simulink model "sampleModel1661"  (R2023a)
settings: Solver=VariableStepAuto  StartTime=0.0  StopTime=10.0  RelTol=1e-3
libraries: hdlsllib x5, simulink x2
settings Model: Creator=user1  LastModifiedBy=user1

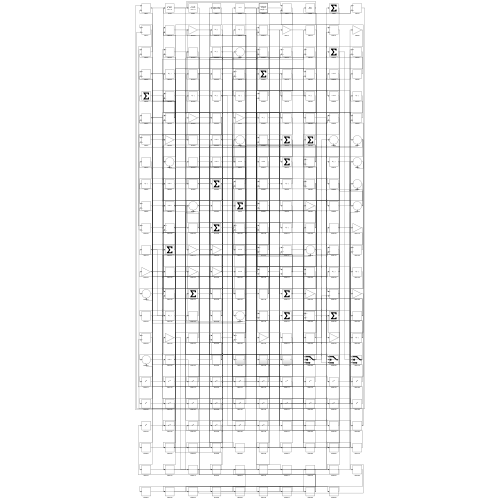
[thumbnail: Simulink's stored preview of the top-level diagram]
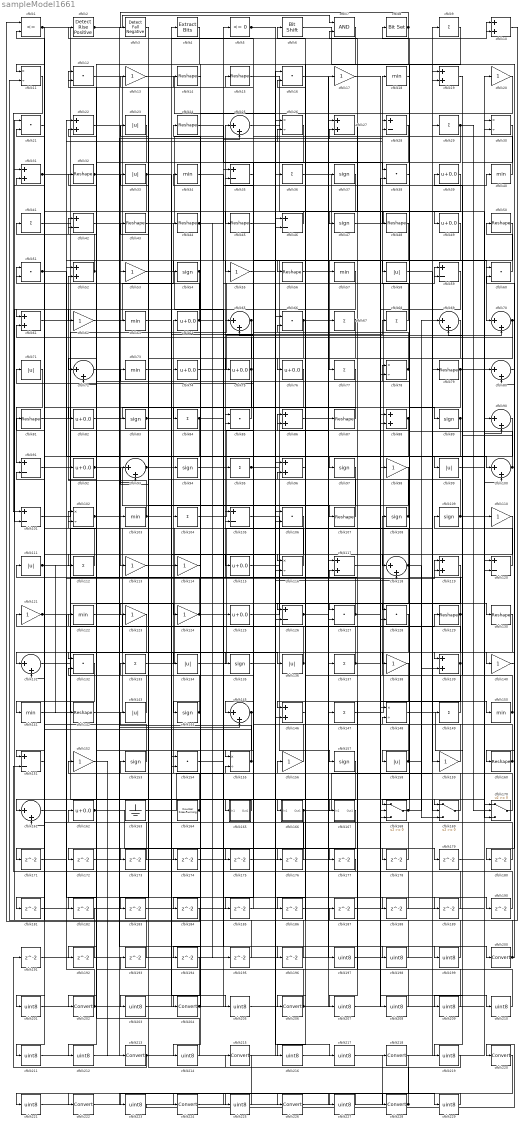
== system sampleModel1661 ==
  cfblk1 : RelationalOperator  Operator=<=  OutDataTypeStr=boolean  InputSameDT=off
  cfblk{10,19,22,27,31,52,61,86,88,96,117,119,139,146} (14 alike) : Sum
  cfblk{25,65,69..70,72,80,90,93,100,118,131,145,161} (13 alike) : Sum  Inputs=|++
  cfblk{28,35,42,46,59,91,101,105,120,126,151} (11 alike) : Sum  Inputs=+-
  cfblk{11,26,30,78,102,116,148,155} (8 alike) : Product  Inputs=*/  RndMeth=Zero  SaturateOnIntegerOverflow=on
  cfblk{18,34,40,57,63,73,103,122,141,150} (10 alike) : MinMax
  cfblk{9,29,36,41,67..68,77,84,95,104,112,133,137,147,149} (15 alike) : Sum  Inputs=+
  cfblk{12,16,21,38,51,60,66,85,106,127..128,132,154} (13 alike) : DotProduct  OutDataTypeStr=Inherit: Inherit via internal rule
  cfblk{14..15,24,32,43..45,48,50,56,79,81,87,107,129..130,142,160} (18 alike) : Reshape
  cfblk{37,47,54,83,89,94,97,108..109,135,144,153,157} (13 alike) : Signum
  cfblk{13,17,20,53,55,62,98,110,113..114,121,123..124,138,140,152,156,159} (18 alike) : Gain
  cfblk{23,33,58,71,99,111,134,136,143,158} (10 alike) : Abs  SaturateOnIntegerOverflow=off
  cfblk{39,49,64,74..76,82,92,115,125,162} (11 alike) : Bias  Bias=0.0  SaturateOnIntegerOverflow=off
  cfblk163 : Ground
  cfblk164 : hdlsllib/Sources/Counter Free-Running  NumBits=16  tsamp=-1
  cfblk165 : Subsystem
      settings: LibrarySourceBlock=|
      | hdlsllib/Ports &
      | Subsystems/Subsystem
  cfblk166 : Subsystem
      settings: LibrarySourceBlock=|
      | hdlsllib/Ports &
      | Subsystems/Subsystem
  cfblk167 : Subsystem
      settings: LibrarySourceBlock=|
      | hdlsllib/Ports &
      | Subsystems/Subsystem
  cfblk168 : Switch  SaturateOnIntegerOverflow=off  InputSameDT=off
  cfblk169 : Switch  SaturateOnIntegerOverflow=off  InputSameDT=off
  cfblk170 : Switch  SaturateOnIntegerOverflow=off  InputSameDT=off
  cfblk{171..196} (26 alike) : Delay  SampleTime=1
  cfblk{197..199,201,203,205,207..212,214,216..217,219,221,223,225,227,229} (21 alike) : DataTypeConversion  OutDataTypeStr=uint8  SaturateOnIntegerOverflow=off  RndMeth=Floor
  cfblk2 : hdlsllib/Logic and Bit Operations/Detect Rise Positive  vinit=0  OutDataTypeStr=boolean
  cfblk{200,202,204,206,213,215,218,220,222,224,226,228} (12 alike) : DataTypeConversion  SaturateOnIntegerOverflow=off  RndMeth=Floor
  cfblk3 : hdlsllib/Logic and Bit Operations/Detect Fall Negative  vinit=0  OutDataTypeStr=boolean
  cfblk4 : simulink/Logic and Bit Operations/Extract Bits  bitsToExtract=Upper half  numBits=8  bitIdxRange=[0 7]  outScalingMode=Preserve fixed-point scaling
      settings: LibrarySourceBlock=|
      | hdlsllib/Logic and Bit
      | Operations/Extract Bits
  cfblk5 : hdlsllib/Logic and Bit Operations/Compare To Zero  relop=<=  OutDataTypeStr=boolean
  cfblk6 : hdlsllib/Logic and Bit Operations/Bit Shift  mode=Shift Left Logical  N=0
  cfblk7 : Logic  AllPortsSameDT=off  OutDataTypeStr=boolean
  cfblk8 : simulink/Logic and Bit Operations/Bit Set  iBit=0
      settings: LibrarySourceBlock=|
      | hdlsllib/Logic and Bit
      | Operations/Bit Set
  wires:
  cfblk147/1 -> cfblk59/1
  cfblk1/1 -> cfblk165/1(In1), cfblk61/1
  cfblk125/1 -> cfblk70/1
  cfblk94/1 -> cfblk200/1
  cfblk169/1 -> cfblk64/1
  cfblk85/1 -> cfblk41/1
  cfblk142/1 -> cfblk104/1
  cfblk68/1 -> cfblk18/1
  cfblk144/1 -> cfblk74/1, cfblk102/1
  cfblk61/1 -> cfblk99/1
  cfblk96/1 -> cfblk166/1(In1)
  cfblk127/1 -> cfblk25/1, cfblk34/1, cfblk169/1
  cfblk101/1 -> cfblk85/1
  cfblk36/1 -> cfblk60/1
  cfblk148/1 -> cfblk162/1
  cfblk82/1 -> cfblk89/1
  cfblk166/1(Out1) -> cfblk29/1, cfblk194/1
  cfblk74/1 -> cfblk70/2
  cfblk6/1 -> cfblk140/1
  cfblk145/1 -> cfblk65/2, cfblk172/1
  cfblk24/1 -> cfblk38/1
  cfblk105/1 -> cfblk157/1
  cfblk49/1 -> cfblk126/1
  cfblk164/1 -> cfblk153/1, cfblk22/2
  cfblk162/1 -> cfblk102/2, cfblk179/1
  cfblk33/1 -> cfblk26/2, cfblk167/1(In1), cfblk171/1
  cfblk104/1 -> cfblk86/1
  cfblk11/1 -> cfblk101/1
  cfblk158/1 -> cfblk71/1, cfblk139/2
  cfblk139/1 -> cfblk15/1, cfblk146/1
  cfblk115/1 -> cfblk127/1
  cfblk133/1 -> cfblk46/1
  cfblk114/1 -> cfblk24/1
  cfblk88/1 -> cfblk86/2, cfblk168/2
  cfblk71/1 -> cfblk91/1
  cfblk120/1 -> cfblk39/1
  cfblk2/1 -> cfblk7/1, cfblk169/2
  cfblk66/1 -> cfblk100/1, cfblk175/1
  cfblk20/1 -> cfblk204/1
  cfblk103/1 -> cfblk52/2, cfblk10/2
  cfblk108/1 -> cfblk35/2, cfblk65/1
  cfblk161/1 -> cfblk119/1
  cfblk37/1 -> cfblk106/2
  cfblk87/1 -> cfblk84/1
  cfblk12/1 -> cfblk55/1
  cfblk41/1 -> cfblk77/1
  cfblk152/1 -> cfblk213/1
  cfblk75/1 -> cfblk141/1, cfblk12/2, cfblk182/1
  cfblk46/1 -> cfblk45/1
  cfblk17/1 -> cfblk150/1
  cfblk111/1 -> cfblk124/1, cfblk142/1
  cfblk22/1 -> cfblk113/1
  cfblk78/1 -> cfblk2/1, cfblk12/1
  cfblk81/1 -> cfblk136/1
  cfblk129/1 -> cfblk73/1, cfblk109/1, cfblk146/2
  cfblk100/1 -> cfblk8/1, cfblk69/2
  cfblk153/1 -> cfblk81/1
  cfblk155/1 -> cfblk143/1, cfblk121/1
  cfblk56/1 -> cfblk87/1
  cfblk95/1 -> cfblk37/1, cfblk217/1
  cfblk25/1 -> cfblk90/2
  cfblk47/1 -> cfblk49/1
  cfblk35/1 -> cfblk145/1
  cfblk44/1 -> cfblk40/1, cfblk195/1
  cfblk116/1 -> cfblk105/1
  cfblk163/1 -> cfblk5/1
  cfblk60/1 -> cfblk50/1
  cfblk90/1 -> cfblk103/1
  cfblk3/1 -> cfblk83/1
  cfblk156/1 -> cfblk133/1
  cfblk135/1 -> cfblk129/1
  cfblk112/1 -> cfblk21/2
  cfblk72/1 -> cfblk27/2
  cfblk113/1 -> cfblk17/1
  cfblk98/1 -> cfblk206/1
  cfblk131/1 -> cfblk105/2
  cfblk13/1 -> cfblk96/1
  cfblk39/1 -> cfblk112/1
  cfblk57/1 -> cfblk144/1
  cfblk58/1 -> cfblk159/1
  cfblk79/1 -> cfblk170/1, cfblk168/1
  cfblk168/1 -> cfblk78/1, cfblk69/1
  cfblk34/1 -> cfblk57/1
  cfblk80/1 -> cfblk160/1
  cfblk43/1 -> cfblk10/1
  cfblk118/1 -> cfblk6/1, cfblk154/2, cfblk169/3
  cfblk134/1 -> cfblk79/1
  cfblk124/1 -> cfblk43/1, cfblk188/1
  cfblk83/1 -> cfblk28/1, cfblk116/2
  cfblk45/1 -> cfblk130/1
  cfblk121/1 -> cfblk38/2, cfblk190/1
  cfblk149/1 -> cfblk108/1
  cfblk160/1 -> cfblk148/2, cfblk111/1
  cfblk170/1 -> cfblk156/1
  cfblk9/1 -> cfblk128/1
  cfblk69/1 -> cfblk76/1
  cfblk42/1 -> cfblk145/2
  cfblk32/1 -> cfblk56/1, cfblk82/1
  cfblk122/1 -> cfblk135/1
  cfblk15/1 -> cfblk48/1
  cfblk67/1 -> cfblk75/1, cfblk116/1
  cfblk126/1 -> cfblk66/2, cfblk198/1
  cfblk65/1 -> cfblk173/1, cfblk174/1
  cfblk28/1 -> cfblk155/1
  cfblk62/1 -> cfblk44/1
  cfblk136/1 -> cfblk122/1, cfblk91/2
  cfblk102/1 -> cfblk93/2, cfblk199/1
  cfblk53/1 -> cfblk95/1
  cfblk54/1 -> cfblk131/1, cfblk101/2
  cfblk38/1 -> cfblk58/1
  cfblk23/1 -> cfblk62/1
  cfblk29/1 -> cfblk63/1, cfblk170/2
  cfblk70/1 -> cfblk78/2, cfblk80/2, cfblk61/2
  cfblk97/1 -> cfblk123/1
  cfblk91/1 -> cfblk36/1
  cfblk59/1 -> cfblk88/2
  cfblk4/1 -> cfblk202/1
  cfblk107/1 -> cfblk13/1
  cfblk165/1(Out1) -> cfblk161/1
  cfblk92/1 -> cfblk125/1, cfblk168/3, cfblk189/1
  cfblk109/1 -> cfblk51/1, cfblk100/2
  cfblk50/1 -> cfblk126/2
  cfblk14/1 -> cfblk134/1
  cfblk137/1 -> cfblk51/2, cfblk210/1
  cfblk5/1 -> cfblk128/2, cfblk118/2
  cfblk130/1 -> cfblk139/1
  cfblk73/1 -> cfblk107/1
  cfblk86/1 -> cfblk67/1
  cfblk89/1 -> cfblk138/1, cfblk158/1
  cfblk52/1 -> cfblk31/2, cfblk42/2
  cfblk27/1 -> cfblk47/1
  cfblk21/1 -> cfblk11/1
  cfblk26/1 -> cfblk72/1
  cfblk31/1 -> cfblk137/1, cfblk28/2
  cfblk99/1 -> cfblk30/2
  cfblk132/1 -> cfblk151/1
  cfblk64/1 -> cfblk42/1, cfblk177/1
  cfblk40/1 -> cfblk14/1
  cfblk141/1 -> cfblk9/1
  cfblk93/1 -> cfblk68/1, cfblk170/3
  cfblk106/1 -> cfblk115/1
  cfblk123/1 -> cfblk132/1
  cfblk8/1 -> cfblk3/1, cfblk214/1
  cfblk159/1 -> cfblk7/2
  cfblk18/1 -> cfblk118/1
  cfblk143/1 -> cfblk92/1
  cfblk84/1 -> cfblk131/2, cfblk196/1
  cfblk51/1 -> cfblk97/1, cfblk54/1
  cfblk150/1 -> cfblk96/2, cfblk119/2
  cfblk154/1 -> cfblk59/2
  cfblk171/1 -> cfblk52/1
  cfblk172/1 -> cfblk35/1
  cfblk173/1 -> cfblk31/1
  cfblk174/1 -> cfblk26/1
  cfblk175/1 -> cfblk27/1
  cfblk7/1 -> cfblk176/1
  cfblk176/1 -> cfblk66/1
  cfblk177/1 -> cfblk151/2
  cfblk55/1 -> cfblk178/1
  cfblk178/1 -> cfblk106/1
  cfblk179/1 -> cfblk90/1
  cfblk140/1 -> cfblk180/1
  cfblk180/1 -> cfblk93/1
  cfblk128/1 -> cfblk181/1
  cfblk181/1 -> cfblk88/1
  cfblk182/1 -> cfblk11/2
  cfblk157/1 -> cfblk183/1
  cfblk183/1 -> cfblk148/1
  cfblk76/1 -> cfblk184/1
  cfblk184/1 -> cfblk1/1
  cfblk48/1 -> cfblk185/1
  cfblk185/1 -> cfblk85/2
  cfblk146/1 -> cfblk186/1
  cfblk186/1 -> cfblk80/1
  cfblk10/1 -> cfblk187/1
  cfblk187/1 -> cfblk120/2
  cfblk188/1 -> cfblk155/2
  cfblk189/1 -> cfblk1/2
  cfblk190/1 -> cfblk72/2
  cfblk191/1 -> cfblk127/2
  cfblk167/1(Out1) -> cfblk192/1
  cfblk192/1 -> cfblk21/1
  cfblk193/1 -> cfblk161/2
  cfblk195/1 -> cfblk23/1
  cfblk196/1 -> cfblk32/1
  cfblk16/1 -> cfblk197/1
  cfblk197/1 -> cfblk149/1
  cfblk198/1 -> cfblk16/1
  cfblk199/1 -> cfblk16/2
  cfblk200/1 -> cfblk60/2, cfblk120/1
  cfblk151/1 -> cfblk201/1
  cfblk201/1 -> cfblk94/1
  cfblk202/1 -> cfblk22/1, cfblk25/2
  cfblk194/1 -> cfblk203/1
  cfblk203/1 -> cfblk4/1
  cfblk204/1 -> cfblk114/1, cfblk147/1
  cfblk63/1 -> cfblk205/1
  cfblk205/1 -> cfblk20/1
  cfblk206/1 -> cfblk132/2, cfblk30/1
  cfblk138/1 -> cfblk207/1
  cfblk207/1 -> cfblk98/1
  cfblk117/1 -> cfblk208/1
  cfblk208/1 -> cfblk154/1
  cfblk30/1 -> cfblk209/1
  cfblk209/1 -> cfblk117/1
  cfblk210/1 -> cfblk117/2
  cfblk110/1 -> cfblk211/1
  cfblk211/1 -> cfblk53/1
  cfblk119/1 -> cfblk212/1
  cfblk212/1 -> cfblk110/1
  cfblk213/1 -> cfblk191/1, cfblk46/2
  cfblk214/1 -> cfblk152/1
  cfblk77/1 -> cfblk216/1
  cfblk216/1 -> cfblk19/1
  cfblk217/1 -> cfblk19/2
  cfblk19/1 -> cfblk219/1
  cfblk219/1 -> cfblk215/1
  cfblk215/1 -> cfblk221/1
  cfblk221/1 -> cfblk218/1
  cfblk218/1 -> cfblk223/1
  cfblk223/1 -> cfblk220/1
  cfblk220/1 -> cfblk225/1
  cfblk225/1 -> cfblk222/1
  cfblk226/1 -> cfblk228/1
  cfblk222/1 -> cfblk227/1
  cfblk227/1 -> cfblk224/1
  cfblk228/1 -> cfblk193/1, cfblk33/1
  cfblk224/1 -> cfblk229/1
  cfblk229/1 -> cfblk226/1

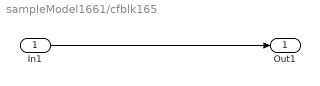
== system sampleModel1661/cfblk165 ==
  In1 : Inport
  Out1 : Outport
  wires:
  In1/1 -> Out1/1

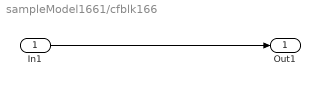
== system sampleModel1661/cfblk166 ==
  In1 : Inport
  Out1 : Outport
  wires:
  In1/1 -> Out1/1

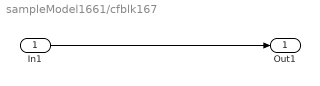
== system sampleModel1661/cfblk167 ==
  In1 : Inport
  Out1 : Outport
  wires:
  In1/1 -> Out1/1
